simulink model "TST_RmtAPP_SelSig"  (R2016b)
settings: Solver=FixedStepDiscrete  StartTime=0.0  StopTime=simTime  FixedStep=sampleTime  RelTol=1e-3
values from neighbouring files (symbols this model uses):
  testCase = 1    [initTST_RmtAPP_SelSig_001.m]    (also in initTST_RmtAPP_SelSig_002.m = 2; initTST_RmtAPP_SelSig_003.m = 3; initTST_RmtAPP_SelSig_004.m = 4)
libraries: simulink x25, UnitTest_Lib x20
settings Model: Creator=liangyunbo  LastModifiedBy=liangyunbo
settings DebuggingCC: SignalRangeChecking=error

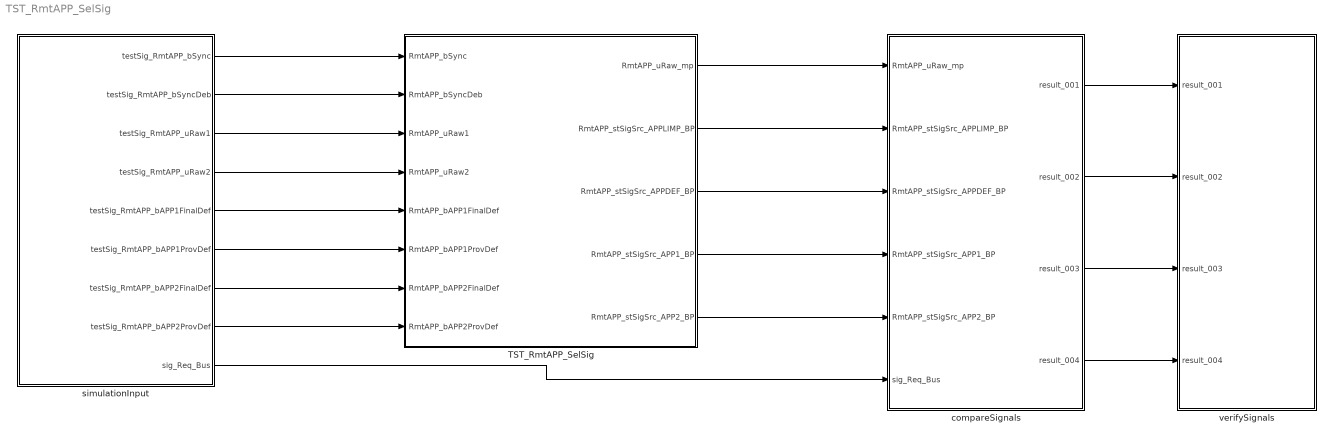
== system TST_RmtAPP_SelSig ==
  TST_RmtAPP_SelSig : Subsystem
  compareSignals : Subsystem
  simulationInput : Subsystem
  verifySignals : Subsystem
  wires:
  simulationInput/1(testSig_RmtAPP_bSync) -> TST_RmtAPP_SelSig/1(RmtAPP_bSync)
  simulationInput/2(testSig_RmtAPP_bSyncDeb) -> TST_RmtAPP_SelSig/2(RmtAPP_bSyncDeb)
  simulationInput/3(testSig_RmtAPP_uRaw1) -> TST_RmtAPP_SelSig/3(RmtAPP_uRaw1)
  simulationInput/4(testSig_RmtAPP_uRaw2) -> TST_RmtAPP_SelSig/4(RmtAPP_uRaw2)
  simulationInput/5(testSig_RmtAPP_bAPP1FinalDef) -> TST_RmtAPP_SelSig/5(RmtAPP_bAPP1FinalDef)
  simulationInput/6(testSig_RmtAPP_bAPP1ProvDef) -> TST_RmtAPP_SelSig/6(RmtAPP_bAPP1ProvDef)
  simulationInput/7(testSig_RmtAPP_bAPP2FinalDef) -> TST_RmtAPP_SelSig/7(RmtAPP_bAPP2FinalDef)
  simulationInput/8(testSig_RmtAPP_bAPP2ProvDef) -> TST_RmtAPP_SelSig/8(RmtAPP_bAPP2ProvDef)
  TST_RmtAPP_SelSig/1(RmtAPP_uRaw_mp) -> compareSignals/1(RmtAPP_uRaw_mp)
  TST_RmtAPP_SelSig/2(RmtAPP_stSigSrc_APPLIMP_BP) -> compareSignals/2(RmtAPP_stSigSrc_APPLIMP_BP)
  TST_RmtAPP_SelSig/3(RmtAPP_stSigSrc_APPDEF_BP) -> compareSignals/3(RmtAPP_stSigSrc_APPDEF_BP)
  TST_RmtAPP_SelSig/4(RmtAPP_stSigSrc_APP1_BP) -> compareSignals/4(RmtAPP_stSigSrc_APP1_BP)
  TST_RmtAPP_SelSig/5(RmtAPP_stSigSrc_APP2_BP) -> compareSignals/5(RmtAPP_stSigSrc_APP2_BP)
  simulationInput/9(sig_Req_Bus) -> compareSignals/6(sig_Req_Bus)
  compareSignals/1(result_001) -> verifySignals/1(result_001)
  compareSignals/2(result_002) -> verifySignals/2(result_002)
  compareSignals/3(result_003) -> verifySignals/3(result_003)
  compareSignals/4(result_004) -> verifySignals/4(result_004)

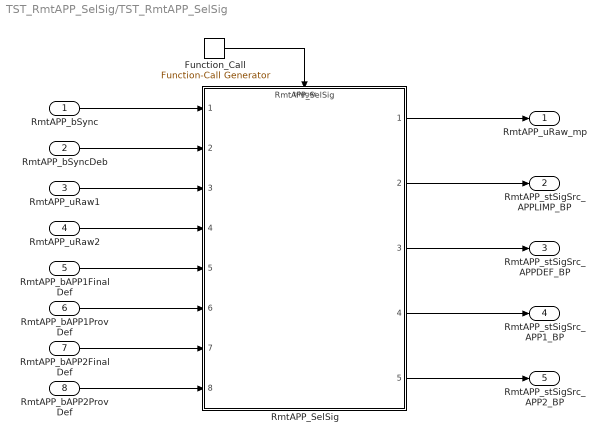
== system TST_RmtAPP_SelSig/TST_RmtAPP_SelSig ==
  RmtAPP_bSync : Inport
  RmtAPP_bSyncDeb : Inport  Port=2
  RmtAPP_uRaw1 : Inport  Port=3
  RmtAPP_uRaw2 : Inport  Port=4
  RmtAPP_bAPP1FinalDef : Inport  Port=5
  RmtAPP_bAPP1ProvDef : Inport  Port=6
  RmtAPP_bAPP2FinalDef : Inport  Port=7
  RmtAPP_bAPP2ProvDef : Inport  Port=8
  Function_Call : simulink/Ports & Subsystems/Function-Call Generator  sample_time=sampleTime  numberOfIterations=1
  RmtAPP_SelSig : ModelReference  ModelNameDialog=RmtAPP_SelSig  SimulationMode=Normal  ModelReferenceVersion=1.6  TriggerPortName=function  TriggerPortTriggerType=function-call  TriggerPortStatesWhenEnabling=held
  RmtAPP_uRaw_mp : Outport
  RmtAPP_stSigSrc_APPLIMP_BP : Outport  Port=2
  RmtAPP_stSigSrc_APPDEF_BP : Outport  Port=3
  RmtAPP_stSigSrc_APP1_BP : Outport  Port=4
  RmtAPP_stSigSrc_APP2_BP : Outport  Port=5
  wires:
  Function_Call/1 -> RmtAPP_SelSig/Trigger
  RmtAPP_bSync/1 -> RmtAPP_SelSig/1
  RmtAPP_bSyncDeb/1 -> RmtAPP_SelSig/2
  RmtAPP_uRaw1/1 -> RmtAPP_SelSig/3
  RmtAPP_uRaw2/1 -> RmtAPP_SelSig/4
  RmtAPP_bAPP1FinalDef/1 -> RmtAPP_SelSig/5
  RmtAPP_bAPP1ProvDef/1 -> RmtAPP_SelSig/6
  RmtAPP_bAPP2FinalDef/1 -> RmtAPP_SelSig/7
  RmtAPP_bAPP2ProvDef/1 -> RmtAPP_SelSig/8
  RmtAPP_SelSig/1 -> RmtAPP_uRaw_mp/1
  RmtAPP_SelSig/2 -> RmtAPP_stSigSrc_APPLIMP_BP/1
  RmtAPP_SelSig/3 -> RmtAPP_stSigSrc_APPDEF_BP/1
  RmtAPP_SelSig/4 -> RmtAPP_stSigSrc_APP1_BP/1
  RmtAPP_SelSig/5 -> RmtAPP_stSigSrc_APP2_BP/1

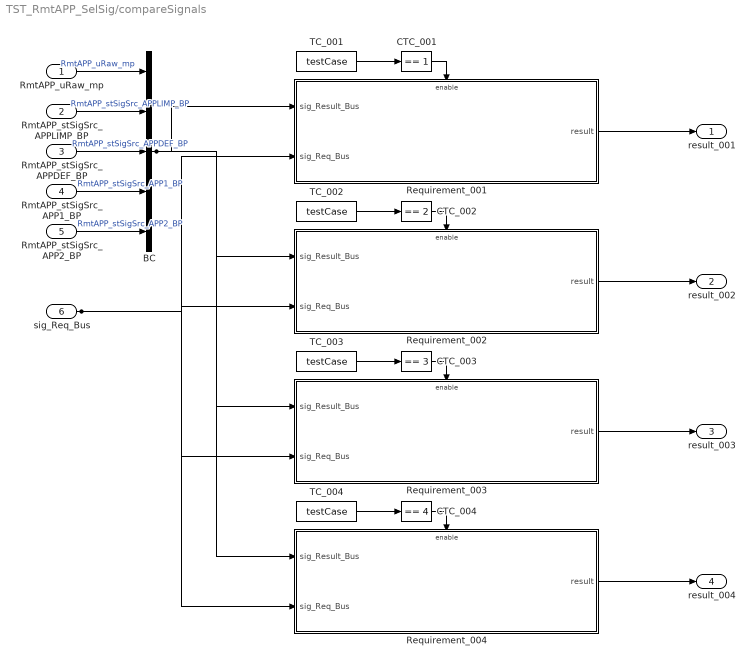
== system TST_RmtAPP_SelSig/compareSignals ==
  RmtAPP_uRaw_mp : Inport
  RmtAPP_stSigSrc_APPLIMP_BP : Inport  Port=2
  RmtAPP_stSigSrc_APPDEF_BP : Inport  Port=3
  RmtAPP_stSigSrc_APP1_BP : Inport  Port=4
  RmtAPP_stSigSrc_APP2_BP : Inport  Port=5
  sig_Req_Bus : Inport  Port=6
  BC : BusCreator  Inputs=5
  CTC_001 : simulink/Logic and Bit Operations/Compare To Constant  relop===  const=1  OutDataTypeStr=boolean
  CTC_002 : simulink/Logic and Bit Operations/Compare To Constant  relop===  const=2  OutDataTypeStr=boolean
  CTC_003 : simulink/Logic and Bit Operations/Compare To Constant  relop===  const=3  OutDataTypeStr=boolean
  CTC_004 : simulink/Logic and Bit Operations/Compare To Constant  relop===  const=4  OutDataTypeStr=boolean
  Requirement_001 : Subsystem
  Requirement_002 : Subsystem
  Requirement_003 : Subsystem
  Requirement_004 : Subsystem
  TC_001 : Constant  Value=testCase
  TC_002 : Constant  Value=testCase
  TC_003 : Constant  Value=testCase
  TC_004 : Constant  Value=testCase
  result_001 : Outport
  result_002 : Outport  Port=2
  result_003 : Outport  Port=3
  result_004 : Outport  Port=4
  wires:
  RmtAPP_uRaw_mp/1 -> BC/1  "RmtAPP_uRaw_mp"
  RmtAPP_stSigSrc_APPLIMP_BP/1 -> BC/2  "RmtAPP_stSigSrc_APPLIMP_BP"
  RmtAPP_stSigSrc_APPDEF_BP/1 -> BC/3  "RmtAPP_stSigSrc_APPDEF_BP"
  RmtAPP_stSigSrc_APP1_BP/1 -> BC/4  "RmtAPP_stSigSrc_APP1_BP"
  RmtAPP_stSigSrc_APP2_BP/1 -> BC/5  "RmtAPP_stSigSrc_APP2_BP"
  TC_001/1 -> CTC_001/1
  CTC_001/1 -> Requirement_001/Enable
  sig_Req_Bus/1 -> Requirement_001/2(sig_Req_Bus), Requirement_002/2(sig_Req_Bus), Requirement_003/2(sig_Req_Bus), Requirement_004/2(sig_Req_Bus)
  BC/1 -> Requirement_001/1(sig_Result_Bus), Requirement_002/1(sig_Result_Bus), Requirement_003/1(sig_Result_Bus), Requirement_004/1(sig_Result_Bus)
  Requirement_001/1(result) -> result_001/1
  TC_002/1 -> CTC_002/1
  CTC_002/1 -> Requirement_002/Enable
  Requirement_002/1(result) -> result_002/1
  TC_003/1 -> CTC_003/1
  CTC_003/1 -> Requirement_003/Enable
  Requirement_003/1(result) -> result_003/1
  TC_004/1 -> CTC_004/1
  CTC_004/1 -> Requirement_004/Enable
  Requirement_004/1(result) -> result_004/1

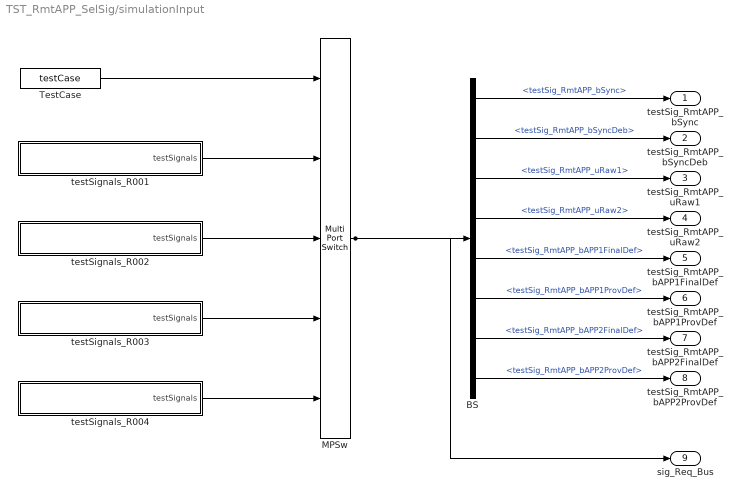
== system TST_RmtAPP_SelSig/simulationInput ==
  BS : BusSelector  OutputSignals=testSig_RmtAPP_bSync,testSig_RmtAPP_bSyncDeb,testSig_RmtAPP_uRaw1,testSig_RmtAPP_uRaw2,testSig_RmtAPP_bAPP1FinalDef,testSig_RmtAPP_bAPP1ProvDef,testSig_RmtAPP_bAPP2FinalDef,testSig_RmtAPP_bAPP2ProvDef
  MPSw : MultiPortSwitch  Inputs=4  SaturateOnIntegerOverflow=on  InputSameDT=on
  TestCase : Constant  Value=testCase
  testSignals_R001 : Subsystem
  testSignals_R002 : Subsystem
  testSignals_R003 : Subsystem
  testSignals_R004 : Subsystem
  testSig_RmtAPP_bSync : Outport
  testSig_RmtAPP_bSyncDeb : Outport  Port=2
  testSig_RmtAPP_uRaw1 : Outport  Port=3
  testSig_RmtAPP_uRaw2 : Outport  Port=4
  testSig_RmtAPP_bAPP1FinalDef : Outport  Port=5
  testSig_RmtAPP_bAPP1ProvDef : Outport  Port=6
  testSig_RmtAPP_bAPP2FinalDef : Outport  Port=7
  testSig_RmtAPP_bAPP2ProvDef : Outport  Port=8
  sig_Req_Bus : Outport  Port=9
  wires:
  BS/1 -> testSig_RmtAPP_bSync/1  "<testSig_RmtAPP_bSync>"
  BS/2 -> testSig_RmtAPP_bSyncDeb/1  "<testSig_RmtAPP_bSyncDeb>"
  BS/3 -> testSig_RmtAPP_uRaw1/1  "<testSig_RmtAPP_uRaw1>"
  BS/4 -> testSig_RmtAPP_uRaw2/1  "<testSig_RmtAPP_uRaw2>"
  BS/5 -> testSig_RmtAPP_bAPP1FinalDef/1  "<testSig_RmtAPP_bAPP1FinalDef>"
  BS/6 -> testSig_RmtAPP_bAPP1ProvDef/1  "<testSig_RmtAPP_bAPP1ProvDef>"
  BS/7 -> testSig_RmtAPP_bAPP2FinalDef/1  "<testSig_RmtAPP_bAPP2FinalDef>"
  BS/8 -> testSig_RmtAPP_bAPP2ProvDef/1  "<testSig_RmtAPP_bAPP2ProvDef>"
  MPSw/1 -> BS/1, sig_Req_Bus/1
  TestCase/1 -> MPSw/1
  testSignals_R001/1(testSignals) -> MPSw/2
  testSignals_R002/1(testSignals) -> MPSw/3
  testSignals_R003/1(testSignals) -> MPSw/4
  testSignals_R004/1(testSignals) -> MPSw/5

== system TST_RmtAPP_SelSig/verifySignals ==
  result_001 : Inport
  result_002 : Inport  Port=2
  result_003 : Inport  Port=3
  result_004 : Inport  Port=4
  Assertion_001 : Assertion  Enabled=off
  Assertion_002 : Assertion  Enabled=off
  Assertion_003 : Assertion  Enabled=off
  Assertion_004 : Assertion  Enabled=off
  wires:
  result_001/1 -> Assertion_001/1
  result_002/1 -> Assertion_002/1
  result_003/1 -> Assertion_003/1
  result_004/1 -> Assertion_004/1

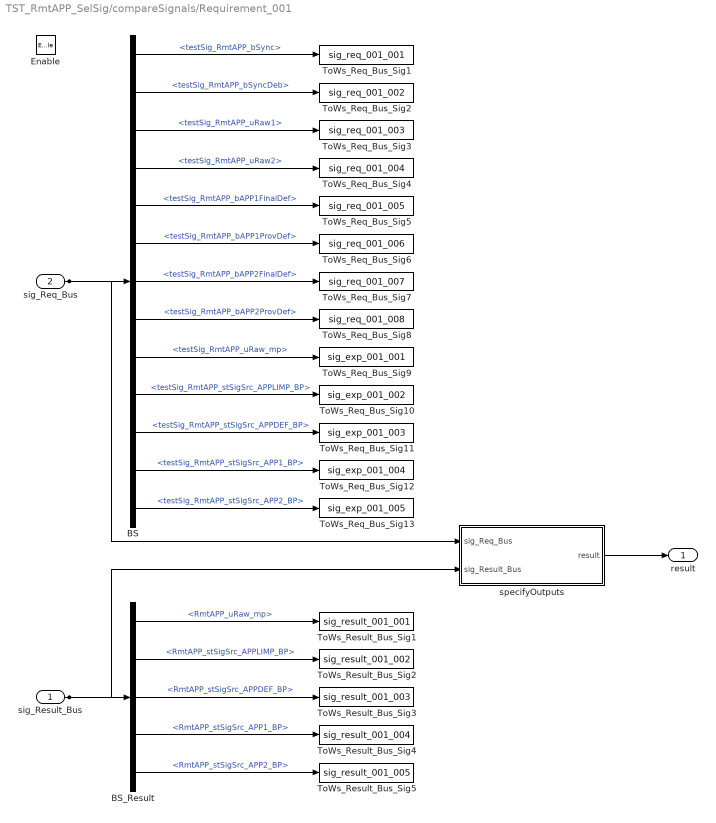
== system TST_RmtAPP_SelSig/compareSignals/Requirement_001 ==
  sig_Result_Bus : Inport
  sig_Req_Bus : Inport  Port=2
  Enable : EnablePort
  BS : BusSelector  OutputSignals=testSig_RmtAPP_bSync,testSig_RmtAPP_bSyncDeb,testSig_RmtAPP_uRaw1,testSig_RmtAPP_uRaw2,testSig_RmtAPP_bAPP1FinalDef,testSig_RmtAPP_bAPP1ProvDef,testSig_RmtAPP_bAPP2FinalDef,testSig_RmtAPP_bAPP2ProvDef,testSig_RmtAPP_uRaw_mp,testSig_RmtAPP_stSigSrc_APPLIMP_BP,testSig_RmtAPP_stSigSrc_APPDEF_BP,testSig_RmtAPP_stSigSrc_APP1_BP,testSig_RmtAPP_stSigSrc_APP2_BP
  BS_Result : BusSelector  OutputSignals=RmtAPP_uRaw_mp,RmtAPP_stSigSrc_APPLIMP_BP,RmtAPP_stSigSrc_APPDEF_BP,RmtAPP_stSigSrc_APP1_BP,RmtAPP_stSigSrc_APP2_BP
  ToWs_Req_Bus_Sig1 : ToWorkspace  VariableName=sig_req_001_001  SaveFormat=Structure With Time
  ToWs_Req_Bus_Sig10 : ToWorkspace  VariableName=sig_exp_001_002  SaveFormat=Structure With Time
  ToWs_Req_Bus_Sig11 : ToWorkspace  VariableName=sig_exp_001_003  SaveFormat=Structure With Time
  ToWs_Req_Bus_Sig12 : ToWorkspace  VariableName=sig_exp_001_004  SaveFormat=Structure With Time
  ToWs_Req_Bus_Sig13 : ToWorkspace  VariableName=sig_exp_001_005  SaveFormat=Structure With Time
  ToWs_Req_Bus_Sig2 : ToWorkspace  VariableName=sig_req_001_002  SaveFormat=Structure With Time
  ToWs_Req_Bus_Sig3 : ToWorkspace  VariableName=sig_req_001_003  SaveFormat=Structure With Time
  ToWs_Req_Bus_Sig4 : ToWorkspace  VariableName=sig_req_001_004  SaveFormat=Structure With Time
  ToWs_Req_Bus_Sig5 : ToWorkspace  VariableName=sig_req_001_005  SaveFormat=Structure With Time
  ToWs_Req_Bus_Sig6 : ToWorkspace  VariableName=sig_req_001_006  SaveFormat=Structure With Time
  ToWs_Req_Bus_Sig7 : ToWorkspace  VariableName=sig_req_001_007  SaveFormat=Structure With Time
  ToWs_Req_Bus_Sig8 : ToWorkspace  VariableName=sig_req_001_008  SaveFormat=Structure With Time
  ToWs_Req_Bus_Sig9 : ToWorkspace  VariableName=sig_exp_001_001  SaveFormat=Structure With Time
  ToWs_Result_Bus_Sig1 : ToWorkspace  VariableName=sig_result_001_001  SaveFormat=Structure With Time
  ToWs_Result_Bus_Sig2 : ToWorkspace  VariableName=sig_result_001_002  SaveFormat=Structure With Time
  ToWs_Result_Bus_Sig3 : ToWorkspace  VariableName=sig_result_001_003  SaveFormat=Structure With Time
  ToWs_Result_Bus_Sig4 : ToWorkspace  VariableName=sig_result_001_004  SaveFormat=Structure With Time
  ToWs_Result_Bus_Sig5 : ToWorkspace  VariableName=sig_result_001_005  SaveFormat=Structure With Time
  specifyOutputs : Subsystem
  result : Outport
  wires:
  sig_Req_Bus/1 -> BS/1, specifyOutputs/1(sig_Req_Bus)
  BS/1 -> ToWs_Req_Bus_Sig1/1  "<testSig_RmtAPP_bSync>"
  BS/2 -> ToWs_Req_Bus_Sig2/1  "<testSig_RmtAPP_bSyncDeb>"
  BS/3 -> ToWs_Req_Bus_Sig3/1  "<testSig_RmtAPP_uRaw1>"
  BS/4 -> ToWs_Req_Bus_Sig4/1  "<testSig_RmtAPP_uRaw2>"
  BS/5 -> ToWs_Req_Bus_Sig5/1  "<testSig_RmtAPP_bAPP1FinalDef>"
  BS/6 -> ToWs_Req_Bus_Sig6/1  "<testSig_RmtAPP_bAPP1ProvDef>"
  BS/7 -> ToWs_Req_Bus_Sig7/1  "<testSig_RmtAPP_bAPP2FinalDef>"
  BS/8 -> ToWs_Req_Bus_Sig8/1  "<testSig_RmtAPP_bAPP2ProvDef>"
  BS/9 -> ToWs_Req_Bus_Sig9/1  "<testSig_RmtAPP_uRaw_mp>"
  BS/10 -> ToWs_Req_Bus_Sig10/1  "<testSig_RmtAPP_stSigSrc_APPLIMP_BP>"
  BS/11 -> ToWs_Req_Bus_Sig11/1  "<testSig_RmtAPP_stSigSrc_APPDEF_BP>"
  BS/12 -> ToWs_Req_Bus_Sig12/1  "<testSig_RmtAPP_stSigSrc_APP1_BP>"
  BS/13 -> ToWs_Req_Bus_Sig13/1  "<testSig_RmtAPP_stSigSrc_APP2_BP>"
  sig_Result_Bus/1 -> BS_Result/1, specifyOutputs/2(sig_Result_Bus)
  BS_Result/1 -> ToWs_Result_Bus_Sig1/1  "<RmtAPP_uRaw_mp>"
  BS_Result/2 -> ToWs_Result_Bus_Sig2/1  "<RmtAPP_stSigSrc_APPLIMP_BP>"
  BS_Result/3 -> ToWs_Result_Bus_Sig3/1  "<RmtAPP_stSigSrc_APPDEF_BP>"
  BS_Result/4 -> ToWs_Result_Bus_Sig4/1  "<RmtAPP_stSigSrc_APP1_BP>"
  BS_Result/5 -> ToWs_Result_Bus_Sig5/1  "<RmtAPP_stSigSrc_APP2_BP>"
  specifyOutputs/1(result) -> result/1

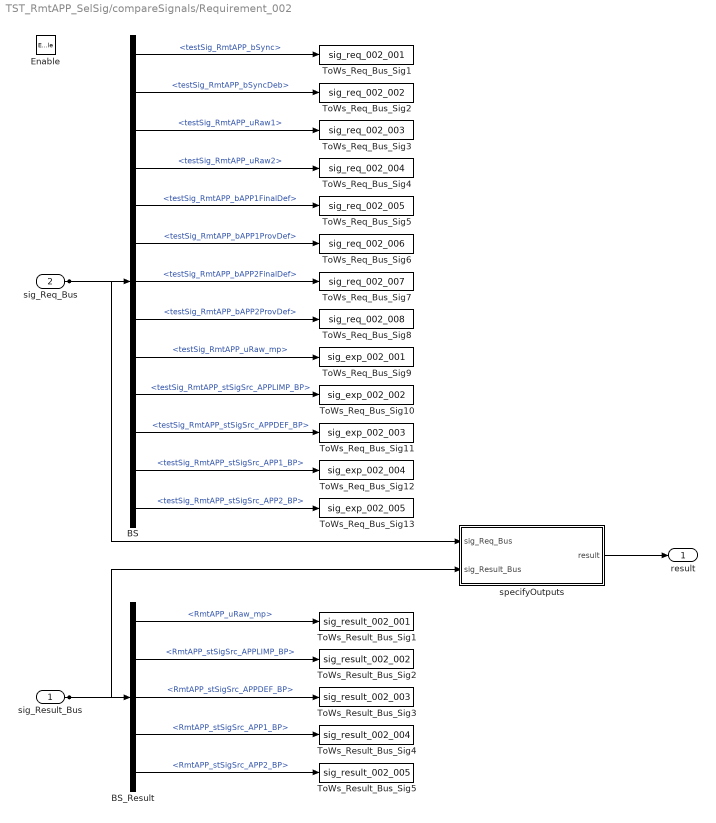
== system TST_RmtAPP_SelSig/compareSignals/Requirement_002 ==
  sig_Result_Bus : Inport
  sig_Req_Bus : Inport  Port=2
  Enable : EnablePort
  BS : BusSelector  OutputSignals=testSig_RmtAPP_bSync,testSig_RmtAPP_bSyncDeb,testSig_RmtAPP_uRaw1,testSig_RmtAPP_uRaw2,testSig_RmtAPP_bAPP1FinalDef,testSig_RmtAPP_bAPP1ProvDef,testSig_RmtAPP_bAPP2FinalDef,testSig_RmtAPP_bAPP2ProvDef,testSig_RmtAPP_uRaw_mp,testSig_RmtAPP_stSigSrc_APPLIMP_BP,testSig_RmtAPP_stSigSrc_APPDEF_BP,testSig_RmtAPP_stSigSrc_APP1_BP,testSig_RmtAPP_stSigSrc_APP2_BP
  BS_Result : BusSelector  OutputSignals=RmtAPP_uRaw_mp,RmtAPP_stSigSrc_APPLIMP_BP,RmtAPP_stSigSrc_APPDEF_BP,RmtAPP_stSigSrc_APP1_BP,RmtAPP_stSigSrc_APP2_BP
  ToWs_Req_Bus_Sig1 : ToWorkspace  VariableName=sig_req_002_001  SaveFormat=Structure With Time
  ToWs_Req_Bus_Sig10 : ToWorkspace  VariableName=sig_exp_002_002  SaveFormat=Structure With Time
  ToWs_Req_Bus_Sig11 : ToWorkspace  VariableName=sig_exp_002_003  SaveFormat=Structure With Time
  ToWs_Req_Bus_Sig12 : ToWorkspace  VariableName=sig_exp_002_004  SaveFormat=Structure With Time
  ToWs_Req_Bus_Sig13 : ToWorkspace  VariableName=sig_exp_002_005  SaveFormat=Structure With Time
  ToWs_Req_Bus_Sig2 : ToWorkspace  VariableName=sig_req_002_002  SaveFormat=Structure With Time
  ToWs_Req_Bus_Sig3 : ToWorkspace  VariableName=sig_req_002_003  SaveFormat=Structure With Time
  ToWs_Req_Bus_Sig4 : ToWorkspace  VariableName=sig_req_002_004  SaveFormat=Structure With Time
  ToWs_Req_Bus_Sig5 : ToWorkspace  VariableName=sig_req_002_005  SaveFormat=Structure With Time
  ToWs_Req_Bus_Sig6 : ToWorkspace  VariableName=sig_req_002_006  SaveFormat=Structure With Time
  ToWs_Req_Bus_Sig7 : ToWorkspace  VariableName=sig_req_002_007  SaveFormat=Structure With Time
  ToWs_Req_Bus_Sig8 : ToWorkspace  VariableName=sig_req_002_008  SaveFormat=Structure With Time
  ToWs_Req_Bus_Sig9 : ToWorkspace  VariableName=sig_exp_002_001  SaveFormat=Structure With Time
  ToWs_Result_Bus_Sig1 : ToWorkspace  VariableName=sig_result_002_001  SaveFormat=Structure With Time
  ToWs_Result_Bus_Sig2 : ToWorkspace  VariableName=sig_result_002_002  SaveFormat=Structure With Time
  ToWs_Result_Bus_Sig3 : ToWorkspace  VariableName=sig_result_002_003  SaveFormat=Structure With Time
  ToWs_Result_Bus_Sig4 : ToWorkspace  VariableName=sig_result_002_004  SaveFormat=Structure With Time
  ToWs_Result_Bus_Sig5 : ToWorkspace  VariableName=sig_result_002_005  SaveFormat=Structure With Time
  specifyOutputs : Subsystem
  result : Outport
  wires:
  sig_Req_Bus/1 -> BS/1, specifyOutputs/1(sig_Req_Bus)
  BS/1 -> ToWs_Req_Bus_Sig1/1  "<testSig_RmtAPP_bSync>"
  BS/2 -> ToWs_Req_Bus_Sig2/1  "<testSig_RmtAPP_bSyncDeb>"
  BS/3 -> ToWs_Req_Bus_Sig3/1  "<testSig_RmtAPP_uRaw1>"
  BS/4 -> ToWs_Req_Bus_Sig4/1  "<testSig_RmtAPP_uRaw2>"
  BS/5 -> ToWs_Req_Bus_Sig5/1  "<testSig_RmtAPP_bAPP1FinalDef>"
  BS/6 -> ToWs_Req_Bus_Sig6/1  "<testSig_RmtAPP_bAPP1ProvDef>"
  BS/7 -> ToWs_Req_Bus_Sig7/1  "<testSig_RmtAPP_bAPP2FinalDef>"
  BS/8 -> ToWs_Req_Bus_Sig8/1  "<testSig_RmtAPP_bAPP2ProvDef>"
  BS/9 -> ToWs_Req_Bus_Sig9/1  "<testSig_RmtAPP_uRaw_mp>"
  BS/10 -> ToWs_Req_Bus_Sig10/1  "<testSig_RmtAPP_stSigSrc_APPLIMP_BP>"
  BS/11 -> ToWs_Req_Bus_Sig11/1  "<testSig_RmtAPP_stSigSrc_APPDEF_BP>"
  BS/12 -> ToWs_Req_Bus_Sig12/1  "<testSig_RmtAPP_stSigSrc_APP1_BP>"
  BS/13 -> ToWs_Req_Bus_Sig13/1  "<testSig_RmtAPP_stSigSrc_APP2_BP>"
  sig_Result_Bus/1 -> BS_Result/1, specifyOutputs/2(sig_Result_Bus)
  BS_Result/1 -> ToWs_Result_Bus_Sig1/1  "<RmtAPP_uRaw_mp>"
  BS_Result/2 -> ToWs_Result_Bus_Sig2/1  "<RmtAPP_stSigSrc_APPLIMP_BP>"
  BS_Result/3 -> ToWs_Result_Bus_Sig3/1  "<RmtAPP_stSigSrc_APPDEF_BP>"
  BS_Result/4 -> ToWs_Result_Bus_Sig4/1  "<RmtAPP_stSigSrc_APP1_BP>"
  BS_Result/5 -> ToWs_Result_Bus_Sig5/1  "<RmtAPP_stSigSrc_APP2_BP>"
  specifyOutputs/1(result) -> result/1

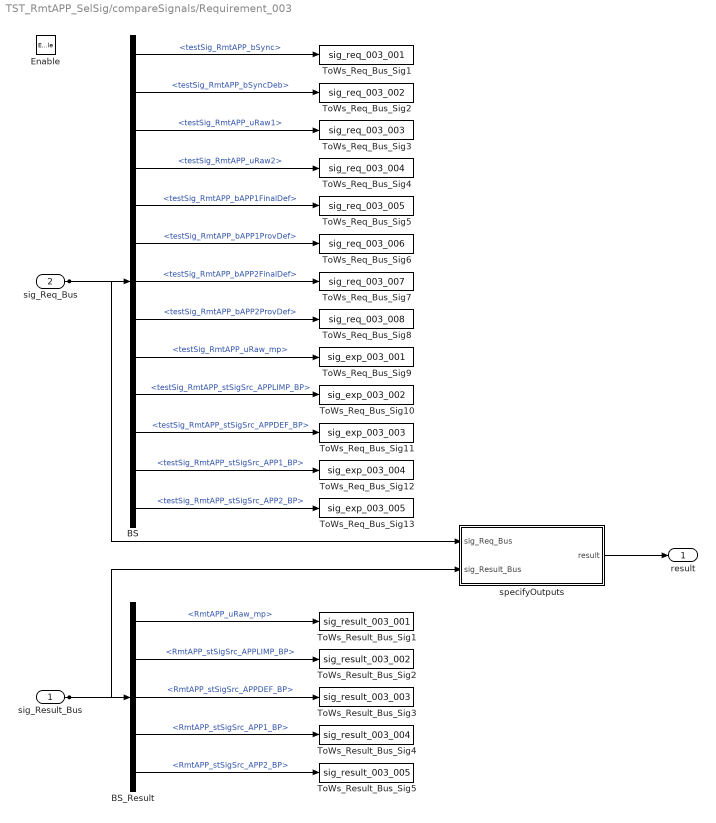
== system TST_RmtAPP_SelSig/compareSignals/Requirement_003 ==
  sig_Result_Bus : Inport
  sig_Req_Bus : Inport  Port=2
  Enable : EnablePort
  BS : BusSelector  OutputSignals=testSig_RmtAPP_bSync,testSig_RmtAPP_bSyncDeb,testSig_RmtAPP_uRaw1,testSig_RmtAPP_uRaw2,testSig_RmtAPP_bAPP1FinalDef,testSig_RmtAPP_bAPP1ProvDef,testSig_RmtAPP_bAPP2FinalDef,testSig_RmtAPP_bAPP2ProvDef,testSig_RmtAPP_uRaw_mp,testSig_RmtAPP_stSigSrc_APPLIMP_BP,testSig_RmtAPP_stSigSrc_APPDEF_BP,testSig_RmtAPP_stSigSrc_APP1_BP,testSig_RmtAPP_stSigSrc_APP2_BP
  BS_Result : BusSelector  OutputSignals=RmtAPP_uRaw_mp,RmtAPP_stSigSrc_APPLIMP_BP,RmtAPP_stSigSrc_APPDEF_BP,RmtAPP_stSigSrc_APP1_BP,RmtAPP_stSigSrc_APP2_BP
  ToWs_Req_Bus_Sig1 : ToWorkspace  VariableName=sig_req_003_001  SaveFormat=Structure With Time
  ToWs_Req_Bus_Sig10 : ToWorkspace  VariableName=sig_exp_003_002  SaveFormat=Structure With Time
  ToWs_Req_Bus_Sig11 : ToWorkspace  VariableName=sig_exp_003_003  SaveFormat=Structure With Time
  ToWs_Req_Bus_Sig12 : ToWorkspace  VariableName=sig_exp_003_004  SaveFormat=Structure With Time
  ToWs_Req_Bus_Sig13 : ToWorkspace  VariableName=sig_exp_003_005  SaveFormat=Structure With Time
  ToWs_Req_Bus_Sig2 : ToWorkspace  VariableName=sig_req_003_002  SaveFormat=Structure With Time
  ToWs_Req_Bus_Sig3 : ToWorkspace  VariableName=sig_req_003_003  SaveFormat=Structure With Time
  ToWs_Req_Bus_Sig4 : ToWorkspace  VariableName=sig_req_003_004  SaveFormat=Structure With Time
  ToWs_Req_Bus_Sig5 : ToWorkspace  VariableName=sig_req_003_005  SaveFormat=Structure With Time
  ToWs_Req_Bus_Sig6 : ToWorkspace  VariableName=sig_req_003_006  SaveFormat=Structure With Time
  ToWs_Req_Bus_Sig7 : ToWorkspace  VariableName=sig_req_003_007  SaveFormat=Structure With Time
  ToWs_Req_Bus_Sig8 : ToWorkspace  VariableName=sig_req_003_008  SaveFormat=Structure With Time
  ToWs_Req_Bus_Sig9 : ToWorkspace  VariableName=sig_exp_003_001  SaveFormat=Structure With Time
  ToWs_Result_Bus_Sig1 : ToWorkspace  VariableName=sig_result_003_001  SaveFormat=Structure With Time
  ToWs_Result_Bus_Sig2 : ToWorkspace  VariableName=sig_result_003_002  SaveFormat=Structure With Time
  ToWs_Result_Bus_Sig3 : ToWorkspace  VariableName=sig_result_003_003  SaveFormat=Structure With Time
  ToWs_Result_Bus_Sig4 : ToWorkspace  VariableName=sig_result_003_004  SaveFormat=Structure With Time
  ToWs_Result_Bus_Sig5 : ToWorkspace  VariableName=sig_result_003_005  SaveFormat=Structure With Time
  specifyOutputs : Subsystem
  result : Outport
  wires:
  sig_Req_Bus/1 -> BS/1, specifyOutputs/1(sig_Req_Bus)
  BS/1 -> ToWs_Req_Bus_Sig1/1  "<testSig_RmtAPP_bSync>"
  BS/2 -> ToWs_Req_Bus_Sig2/1  "<testSig_RmtAPP_bSyncDeb>"
  BS/3 -> ToWs_Req_Bus_Sig3/1  "<testSig_RmtAPP_uRaw1>"
  BS/4 -> ToWs_Req_Bus_Sig4/1  "<testSig_RmtAPP_uRaw2>"
  BS/5 -> ToWs_Req_Bus_Sig5/1  "<testSig_RmtAPP_bAPP1FinalDef>"
  BS/6 -> ToWs_Req_Bus_Sig6/1  "<testSig_RmtAPP_bAPP1ProvDef>"
  BS/7 -> ToWs_Req_Bus_Sig7/1  "<testSig_RmtAPP_bAPP2FinalDef>"
  BS/8 -> ToWs_Req_Bus_Sig8/1  "<testSig_RmtAPP_bAPP2ProvDef>"
  BS/9 -> ToWs_Req_Bus_Sig9/1  "<testSig_RmtAPP_uRaw_mp>"
  BS/10 -> ToWs_Req_Bus_Sig10/1  "<testSig_RmtAPP_stSigSrc_APPLIMP_BP>"
  BS/11 -> ToWs_Req_Bus_Sig11/1  "<testSig_RmtAPP_stSigSrc_APPDEF_BP>"
  BS/12 -> ToWs_Req_Bus_Sig12/1  "<testSig_RmtAPP_stSigSrc_APP1_BP>"
  BS/13 -> ToWs_Req_Bus_Sig13/1  "<testSig_RmtAPP_stSigSrc_APP2_BP>"
  sig_Result_Bus/1 -> BS_Result/1, specifyOutputs/2(sig_Result_Bus)
  BS_Result/1 -> ToWs_Result_Bus_Sig1/1  "<RmtAPP_uRaw_mp>"
  BS_Result/2 -> ToWs_Result_Bus_Sig2/1  "<RmtAPP_stSigSrc_APPLIMP_BP>"
  BS_Result/3 -> ToWs_Result_Bus_Sig3/1  "<RmtAPP_stSigSrc_APPDEF_BP>"
  BS_Result/4 -> ToWs_Result_Bus_Sig4/1  "<RmtAPP_stSigSrc_APP1_BP>"
  BS_Result/5 -> ToWs_Result_Bus_Sig5/1  "<RmtAPP_stSigSrc_APP2_BP>"
  specifyOutputs/1(result) -> result/1

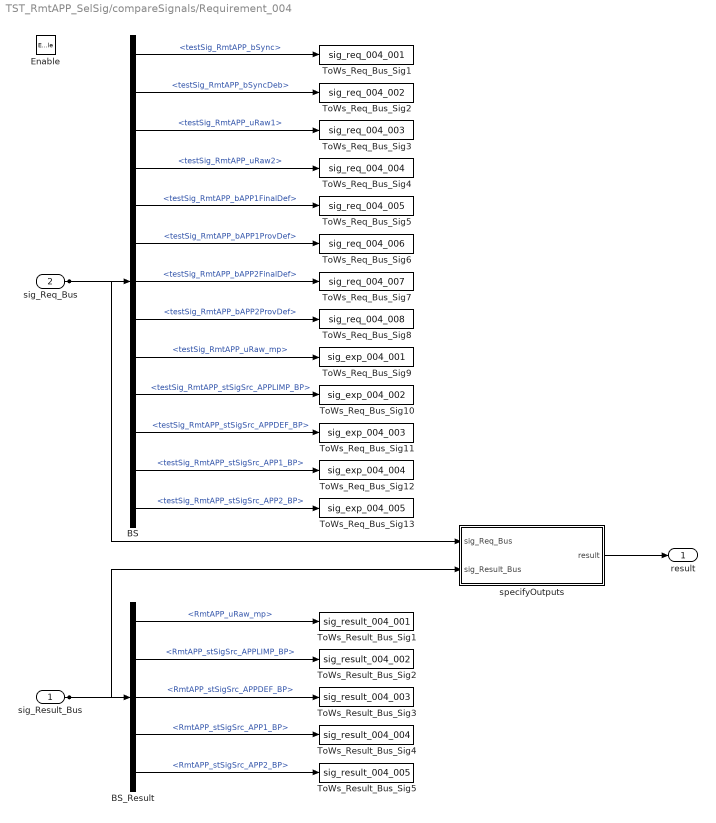
== system TST_RmtAPP_SelSig/compareSignals/Requirement_004 ==
  sig_Result_Bus : Inport
  sig_Req_Bus : Inport  Port=2
  Enable : EnablePort
  BS : BusSelector  OutputSignals=testSig_RmtAPP_bSync,testSig_RmtAPP_bSyncDeb,testSig_RmtAPP_uRaw1,testSig_RmtAPP_uRaw2,testSig_RmtAPP_bAPP1FinalDef,testSig_RmtAPP_bAPP1ProvDef,testSig_RmtAPP_bAPP2FinalDef,testSig_RmtAPP_bAPP2ProvDef,testSig_RmtAPP_uRaw_mp,testSig_RmtAPP_stSigSrc_APPLIMP_BP,testSig_RmtAPP_stSigSrc_APPDEF_BP,testSig_RmtAPP_stSigSrc_APP1_BP,testSig_RmtAPP_stSigSrc_APP2_BP
  BS_Result : BusSelector  OutputSignals=RmtAPP_uRaw_mp,RmtAPP_stSigSrc_APPLIMP_BP,RmtAPP_stSigSrc_APPDEF_BP,RmtAPP_stSigSrc_APP1_BP,RmtAPP_stSigSrc_APP2_BP
  ToWs_Req_Bus_Sig1 : ToWorkspace  VariableName=sig_req_004_001  SaveFormat=Structure With Time
  ToWs_Req_Bus_Sig10 : ToWorkspace  VariableName=sig_exp_004_002  SaveFormat=Structure With Time
  ToWs_Req_Bus_Sig11 : ToWorkspace  VariableName=sig_exp_004_003  SaveFormat=Structure With Time
  ToWs_Req_Bus_Sig12 : ToWorkspace  VariableName=sig_exp_004_004  SaveFormat=Structure With Time
  ToWs_Req_Bus_Sig13 : ToWorkspace  VariableName=sig_exp_004_005  SaveFormat=Structure With Time
  ToWs_Req_Bus_Sig2 : ToWorkspace  VariableName=sig_req_004_002  SaveFormat=Structure With Time
  ToWs_Req_Bus_Sig3 : ToWorkspace  VariableName=sig_req_004_003  SaveFormat=Structure With Time
  ToWs_Req_Bus_Sig4 : ToWorkspace  VariableName=sig_req_004_004  SaveFormat=Structure With Time
  ToWs_Req_Bus_Sig5 : ToWorkspace  VariableName=sig_req_004_005  SaveFormat=Structure With Time
  ToWs_Req_Bus_Sig6 : ToWorkspace  VariableName=sig_req_004_006  SaveFormat=Structure With Time
  ToWs_Req_Bus_Sig7 : ToWorkspace  VariableName=sig_req_004_007  SaveFormat=Structure With Time
  ToWs_Req_Bus_Sig8 : ToWorkspace  VariableName=sig_req_004_008  SaveFormat=Structure With Time
  ToWs_Req_Bus_Sig9 : ToWorkspace  VariableName=sig_exp_004_001  SaveFormat=Structure With Time
  ToWs_Result_Bus_Sig1 : ToWorkspace  VariableName=sig_result_004_001  SaveFormat=Structure With Time
  ToWs_Result_Bus_Sig2 : ToWorkspace  VariableName=sig_result_004_002  SaveFormat=Structure With Time
  ToWs_Result_Bus_Sig3 : ToWorkspace  VariableName=sig_result_004_003  SaveFormat=Structure With Time
  ToWs_Result_Bus_Sig4 : ToWorkspace  VariableName=sig_result_004_004  SaveFormat=Structure With Time
  ToWs_Result_Bus_Sig5 : ToWorkspace  VariableName=sig_result_004_005  SaveFormat=Structure With Time
  specifyOutputs : Subsystem
  result : Outport
  wires:
  sig_Req_Bus/1 -> BS/1, specifyOutputs/1(sig_Req_Bus)
  BS/1 -> ToWs_Req_Bus_Sig1/1  "<testSig_RmtAPP_bSync>"
  BS/2 -> ToWs_Req_Bus_Sig2/1  "<testSig_RmtAPP_bSyncDeb>"
  BS/3 -> ToWs_Req_Bus_Sig3/1  "<testSig_RmtAPP_uRaw1>"
  BS/4 -> ToWs_Req_Bus_Sig4/1  "<testSig_RmtAPP_uRaw2>"
  BS/5 -> ToWs_Req_Bus_Sig5/1  "<testSig_RmtAPP_bAPP1FinalDef>"
  BS/6 -> ToWs_Req_Bus_Sig6/1  "<testSig_RmtAPP_bAPP1ProvDef>"
  BS/7 -> ToWs_Req_Bus_Sig7/1  "<testSig_RmtAPP_bAPP2FinalDef>"
  BS/8 -> ToWs_Req_Bus_Sig8/1  "<testSig_RmtAPP_bAPP2ProvDef>"
  BS/9 -> ToWs_Req_Bus_Sig9/1  "<testSig_RmtAPP_uRaw_mp>"
  BS/10 -> ToWs_Req_Bus_Sig10/1  "<testSig_RmtAPP_stSigSrc_APPLIMP_BP>"
  BS/11 -> ToWs_Req_Bus_Sig11/1  "<testSig_RmtAPP_stSigSrc_APPDEF_BP>"
  BS/12 -> ToWs_Req_Bus_Sig12/1  "<testSig_RmtAPP_stSigSrc_APP1_BP>"
  BS/13 -> ToWs_Req_Bus_Sig13/1  "<testSig_RmtAPP_stSigSrc_APP2_BP>"
  sig_Result_Bus/1 -> BS_Result/1, specifyOutputs/2(sig_Result_Bus)
  BS_Result/1 -> ToWs_Result_Bus_Sig1/1  "<RmtAPP_uRaw_mp>"
  BS_Result/2 -> ToWs_Result_Bus_Sig2/1  "<RmtAPP_stSigSrc_APPLIMP_BP>"
  BS_Result/3 -> ToWs_Result_Bus_Sig3/1  "<RmtAPP_stSigSrc_APPDEF_BP>"
  BS_Result/4 -> ToWs_Result_Bus_Sig4/1  "<RmtAPP_stSigSrc_APP1_BP>"
  BS_Result/5 -> ToWs_Result_Bus_Sig5/1  "<RmtAPP_stSigSrc_APP2_BP>"
  specifyOutputs/1(result) -> result/1

== system TST_RmtAPP_SelSig/simulationInput/testSignals_R001 ==
  BC : BusCreator  Inputs=13
  spec_RmtAPP_bAPP1FinalDef : FromWorkspace  VariableName=testSig_RmtAPP_bAPP1FinalDef  Interpolate=off  OutputAfterFinalValue=Holding final value
  spec_RmtAPP_bAPP1ProvDef : FromWorkspace  VariableName=testSig_RmtAPP_bAPP1ProvDef  Interpolate=off  OutputAfterFinalValue=Holding final value
  spec_RmtAPP_bAPP2FinalDef : FromWorkspace  VariableName=testSig_RmtAPP_bAPP2FinalDef  Interpolate=off  OutputAfterFinalValue=Holding final value
  spec_RmtAPP_bAPP2ProvDef : FromWorkspace  VariableName=testSig_RmtAPP_bAPP2ProvDef  Interpolate=off  OutputAfterFinalValue=Holding final value
  spec_RmtAPP_bSync : FromWorkspace  VariableName=testSig_RmtAPP_bSync  Interpolate=off  OutputAfterFinalValue=Holding final value
  spec_RmtAPP_bSyncDeb : FromWorkspace  VariableName=testSig_RmtAPP_bSyncDeb  Interpolate=off  OutputAfterFinalValue=Holding final value
  spec_RmtAPP_stSigSrc_APP1_BP : FromWorkspace  VariableName=testSig_RmtAPP_stSigSrc_APP1_BP  Interpolate=off  OutputAfterFinalValue=Holding final value
  spec_RmtAPP_stSigSrc_APP2_BP : FromWorkspace  VariableName=testSig_RmtAPP_stSigSrc_APP2_BP  Interpolate=off  OutputAfterFinalValue=Holding final value
  spec_RmtAPP_stSigSrc_APPDEF_BP : FromWorkspace  VariableName=testSig_RmtAPP_stSigSrc_APPDEF_BP  Interpolate=off  OutputAfterFinalValue=Holding final value
  spec_RmtAPP_stSigSrc_APPLIMP_BP : FromWorkspace  VariableName=testSig_RmtAPP_stSigSrc_APPLIMP_BP  Interpolate=off  OutputAfterFinalValue=Holding final value
  spec_RmtAPP_uRaw1 : FromWorkspace  VariableName=testSig_RmtAPP_uRaw1  Interpolate=off  OutputAfterFinalValue=Holding final value
  spec_RmtAPP_uRaw2 : FromWorkspace  VariableName=testSig_RmtAPP_uRaw2  Interpolate=off  OutputAfterFinalValue=Holding final value
  spec_RmtAPP_uRaw_mp : FromWorkspace  VariableName=testSig_RmtAPP_uRaw_mp  Interpolate=off  OutputAfterFinalValue=Holding final value
  testSignals : Outport
  wires:
  BC/1 -> testSignals/1
  spec_RmtAPP_bSync/1 -> BC/1  "testSig_RmtAPP_bSync"
  spec_RmtAPP_bSyncDeb/1 -> BC/2  "testSig_RmtAPP_bSyncDeb"
  spec_RmtAPP_uRaw1/1 -> BC/3  "testSig_RmtAPP_uRaw1"
  spec_RmtAPP_uRaw2/1 -> BC/4  "testSig_RmtAPP_uRaw2"
  spec_RmtAPP_bAPP1FinalDef/1 -> BC/5  "testSig_RmtAPP_bAPP1FinalDef"
  spec_RmtAPP_bAPP1ProvDef/1 -> BC/6  "testSig_RmtAPP_bAPP1ProvDef"
  spec_RmtAPP_bAPP2FinalDef/1 -> BC/7  "testSig_RmtAPP_bAPP2FinalDef"
  spec_RmtAPP_bAPP2ProvDef/1 -> BC/8  "testSig_RmtAPP_bAPP2ProvDef"
  spec_RmtAPP_uRaw_mp/1 -> BC/9  "testSig_RmtAPP_uRaw_mp"
  spec_RmtAPP_stSigSrc_APPLIMP_BP/1 -> BC/10  "testSig_RmtAPP_stSigSrc_APPLIMP_BP"
  spec_RmtAPP_stSigSrc_APPDEF_BP/1 -> BC/11  "testSig_RmtAPP_stSigSrc_APPDEF_BP"
  spec_RmtAPP_stSigSrc_APP1_BP/1 -> BC/12  "testSig_RmtAPP_stSigSrc_APP1_BP"
  spec_RmtAPP_stSigSrc_APP2_BP/1 -> BC/13  "testSig_RmtAPP_stSigSrc_APP2_BP"

== system TST_RmtAPP_SelSig/simulationInput/testSignals_R002 ==
  BC : BusCreator  Inputs=13
  spec_RmtAPP_bAPP1FinalDef : FromWorkspace  VariableName=testSig_RmtAPP_bAPP1FinalDef  Interpolate=off  OutputAfterFinalValue=Holding final value
  spec_RmtAPP_bAPP1ProvDef : FromWorkspace  VariableName=testSig_RmtAPP_bAPP1ProvDef  Interpolate=off  OutputAfterFinalValue=Holding final value
  spec_RmtAPP_bAPP2FinalDef : FromWorkspace  VariableName=testSig_RmtAPP_bAPP2FinalDef  Interpolate=off  OutputAfterFinalValue=Holding final value
  spec_RmtAPP_bAPP2ProvDef : FromWorkspace  VariableName=testSig_RmtAPP_bAPP2ProvDef  Interpolate=off  OutputAfterFinalValue=Holding final value
  spec_RmtAPP_bSync : FromWorkspace  VariableName=testSig_RmtAPP_bSync  Interpolate=off  OutputAfterFinalValue=Holding final value
  spec_RmtAPP_bSyncDeb : FromWorkspace  VariableName=testSig_RmtAPP_bSyncDeb  Interpolate=off  OutputAfterFinalValue=Holding final value
  spec_RmtAPP_stSigSrc_APP1_BP : FromWorkspace  VariableName=testSig_RmtAPP_stSigSrc_APP1_BP  Interpolate=off  OutputAfterFinalValue=Holding final value
  spec_RmtAPP_stSigSrc_APP2_BP : FromWorkspace  VariableName=testSig_RmtAPP_stSigSrc_APP2_BP  Interpolate=off  OutputAfterFinalValue=Holding final value
  spec_RmtAPP_stSigSrc_APPDEF_BP : FromWorkspace  VariableName=testSig_RmtAPP_stSigSrc_APPDEF_BP  Interpolate=off  OutputAfterFinalValue=Holding final value
  spec_RmtAPP_stSigSrc_APPLIMP_BP : FromWorkspace  VariableName=testSig_RmtAPP_stSigSrc_APPLIMP_BP  Interpolate=off  OutputAfterFinalValue=Holding final value
  spec_RmtAPP_uRaw1 : FromWorkspace  VariableName=testSig_RmtAPP_uRaw1  Interpolate=off  OutputAfterFinalValue=Holding final value
  spec_RmtAPP_uRaw2 : FromWorkspace  VariableName=testSig_RmtAPP_uRaw2  Interpolate=off  OutputAfterFinalValue=Holding final value
  spec_RmtAPP_uRaw_mp : FromWorkspace  VariableName=testSig_RmtAPP_uRaw_mp  Interpolate=off  OutputAfterFinalValue=Holding final value
  testSignals : Outport
  wires:
  BC/1 -> testSignals/1
  spec_RmtAPP_bSync/1 -> BC/1  "testSig_RmtAPP_bSync"
  spec_RmtAPP_bSyncDeb/1 -> BC/2  "testSig_RmtAPP_bSyncDeb"
  spec_RmtAPP_uRaw1/1 -> BC/3  "testSig_RmtAPP_uRaw1"
  spec_RmtAPP_uRaw2/1 -> BC/4  "testSig_RmtAPP_uRaw2"
  spec_RmtAPP_bAPP1FinalDef/1 -> BC/5  "testSig_RmtAPP_bAPP1FinalDef"
  spec_RmtAPP_bAPP1ProvDef/1 -> BC/6  "testSig_RmtAPP_bAPP1ProvDef"
  spec_RmtAPP_bAPP2FinalDef/1 -> BC/7  "testSig_RmtAPP_bAPP2FinalDef"
  spec_RmtAPP_bAPP2ProvDef/1 -> BC/8  "testSig_RmtAPP_bAPP2ProvDef"
  spec_RmtAPP_uRaw_mp/1 -> BC/9  "testSig_RmtAPP_uRaw_mp"
  spec_RmtAPP_stSigSrc_APPLIMP_BP/1 -> BC/10  "testSig_RmtAPP_stSigSrc_APPLIMP_BP"
  spec_RmtAPP_stSigSrc_APPDEF_BP/1 -> BC/11  "testSig_RmtAPP_stSigSrc_APPDEF_BP"
  spec_RmtAPP_stSigSrc_APP1_BP/1 -> BC/12  "testSig_RmtAPP_stSigSrc_APP1_BP"
  spec_RmtAPP_stSigSrc_APP2_BP/1 -> BC/13  "testSig_RmtAPP_stSigSrc_APP2_BP"

== system TST_RmtAPP_SelSig/simulationInput/testSignals_R003 ==
  BC : BusCreator  Inputs=13
  spec_RmtAPP_bAPP1FinalDef : FromWorkspace  VariableName=testSig_RmtAPP_bAPP1FinalDef  Interpolate=off  OutputAfterFinalValue=Holding final value
  spec_RmtAPP_bAPP1ProvDef : FromWorkspace  VariableName=testSig_RmtAPP_bAPP1ProvDef  Interpolate=off  OutputAfterFinalValue=Holding final value
  spec_RmtAPP_bAPP2FinalDef : FromWorkspace  VariableName=testSig_RmtAPP_bAPP2FinalDef  Interpolate=off  OutputAfterFinalValue=Holding final value
  spec_RmtAPP_bAPP2ProvDef : FromWorkspace  VariableName=testSig_RmtAPP_bAPP2ProvDef  Interpolate=off  OutputAfterFinalValue=Holding final value
  spec_RmtAPP_bSync : FromWorkspace  VariableName=testSig_RmtAPP_bSync  Interpolate=off  OutputAfterFinalValue=Holding final value
  spec_RmtAPP_bSyncDeb : FromWorkspace  VariableName=testSig_RmtAPP_bSyncDeb  Interpolate=off  OutputAfterFinalValue=Holding final value
  spec_RmtAPP_stSigSrc_APP1_BP : FromWorkspace  VariableName=testSig_RmtAPP_stSigSrc_APP1_BP  Interpolate=off  OutputAfterFinalValue=Holding final value
  spec_RmtAPP_stSigSrc_APP2_BP : FromWorkspace  VariableName=testSig_RmtAPP_stSigSrc_APP2_BP  Interpolate=off  OutputAfterFinalValue=Holding final value
  spec_RmtAPP_stSigSrc_APPDEF_BP : FromWorkspace  VariableName=testSig_RmtAPP_stSigSrc_APPDEF_BP  Interpolate=off  OutputAfterFinalValue=Holding final value
  spec_RmtAPP_stSigSrc_APPLIMP_BP : FromWorkspace  VariableName=testSig_RmtAPP_stSigSrc_APPLIMP_BP  Interpolate=off  OutputAfterFinalValue=Holding final value
  spec_RmtAPP_uRaw1 : FromWorkspace  VariableName=testSig_RmtAPP_uRaw1  Interpolate=off  OutputAfterFinalValue=Holding final value
  spec_RmtAPP_uRaw2 : FromWorkspace  VariableName=testSig_RmtAPP_uRaw2  Interpolate=off  OutputAfterFinalValue=Holding final value
  spec_RmtAPP_uRaw_mp : FromWorkspace  VariableName=testSig_RmtAPP_uRaw_mp  Interpolate=off  OutputAfterFinalValue=Holding final value
  testSignals : Outport
  wires:
  BC/1 -> testSignals/1
  spec_RmtAPP_bSync/1 -> BC/1  "testSig_RmtAPP_bSync"
  spec_RmtAPP_bSyncDeb/1 -> BC/2  "testSig_RmtAPP_bSyncDeb"
  spec_RmtAPP_uRaw1/1 -> BC/3  "testSig_RmtAPP_uRaw1"
  spec_RmtAPP_uRaw2/1 -> BC/4  "testSig_RmtAPP_uRaw2"
  spec_RmtAPP_bAPP1FinalDef/1 -> BC/5  "testSig_RmtAPP_bAPP1FinalDef"
  spec_RmtAPP_bAPP1ProvDef/1 -> BC/6  "testSig_RmtAPP_bAPP1ProvDef"
  spec_RmtAPP_bAPP2FinalDef/1 -> BC/7  "testSig_RmtAPP_bAPP2FinalDef"
  spec_RmtAPP_bAPP2ProvDef/1 -> BC/8  "testSig_RmtAPP_bAPP2ProvDef"
  spec_RmtAPP_uRaw_mp/1 -> BC/9  "testSig_RmtAPP_uRaw_mp"
  spec_RmtAPP_stSigSrc_APPLIMP_BP/1 -> BC/10  "testSig_RmtAPP_stSigSrc_APPLIMP_BP"
  spec_RmtAPP_stSigSrc_APPDEF_BP/1 -> BC/11  "testSig_RmtAPP_stSigSrc_APPDEF_BP"
  spec_RmtAPP_stSigSrc_APP1_BP/1 -> BC/12  "testSig_RmtAPP_stSigSrc_APP1_BP"
  spec_RmtAPP_stSigSrc_APP2_BP/1 -> BC/13  "testSig_RmtAPP_stSigSrc_APP2_BP"

== system TST_RmtAPP_SelSig/simulationInput/testSignals_R004 ==
  BC : BusCreator  Inputs=13
  spec_RmtAPP_bAPP1FinalDef : FromWorkspace  VariableName=testSig_RmtAPP_bAPP1FinalDef  Interpolate=off  OutputAfterFinalValue=Holding final value
  spec_RmtAPP_bAPP1ProvDef : FromWorkspace  VariableName=testSig_RmtAPP_bAPP1ProvDef  Interpolate=off  OutputAfterFinalValue=Holding final value
  spec_RmtAPP_bAPP2FinalDef : FromWorkspace  VariableName=testSig_RmtAPP_bAPP2FinalDef  Interpolate=off  OutputAfterFinalValue=Holding final value
  spec_RmtAPP_bAPP2ProvDef : FromWorkspace  VariableName=testSig_RmtAPP_bAPP2ProvDef  Interpolate=off  OutputAfterFinalValue=Holding final value
  spec_RmtAPP_bSync : FromWorkspace  VariableName=testSig_RmtAPP_bSync  Interpolate=off  OutputAfterFinalValue=Holding final value
  spec_RmtAPP_bSyncDeb : FromWorkspace  VariableName=testSig_RmtAPP_bSyncDeb  Interpolate=off  OutputAfterFinalValue=Holding final value
  spec_RmtAPP_stSigSrc_APP1_BP : FromWorkspace  VariableName=testSig_RmtAPP_stSigSrc_APP1_BP  Interpolate=off  OutputAfterFinalValue=Holding final value
  spec_RmtAPP_stSigSrc_APP2_BP : FromWorkspace  VariableName=testSig_RmtAPP_stSigSrc_APP2_BP  Interpolate=off  OutputAfterFinalValue=Holding final value
  spec_RmtAPP_stSigSrc_APPDEF_BP : FromWorkspace  VariableName=testSig_RmtAPP_stSigSrc_APPDEF_BP  Interpolate=off  OutputAfterFinalValue=Holding final value
  spec_RmtAPP_stSigSrc_APPLIMP_BP : FromWorkspace  VariableName=testSig_RmtAPP_stSigSrc_APPLIMP_BP  Interpolate=off  OutputAfterFinalValue=Holding final value
  spec_RmtAPP_uRaw1 : FromWorkspace  VariableName=testSig_RmtAPP_uRaw1  Interpolate=off  OutputAfterFinalValue=Holding final value
  spec_RmtAPP_uRaw2 : FromWorkspace  VariableName=testSig_RmtAPP_uRaw2  Interpolate=off  OutputAfterFinalValue=Holding final value
  spec_RmtAPP_uRaw_mp : FromWorkspace  VariableName=testSig_RmtAPP_uRaw_mp  Interpolate=off  OutputAfterFinalValue=Holding final value
  testSignals : Outport
  wires:
  BC/1 -> testSignals/1
  spec_RmtAPP_bSync/1 -> BC/1  "testSig_RmtAPP_bSync"
  spec_RmtAPP_bSyncDeb/1 -> BC/2  "testSig_RmtAPP_bSyncDeb"
  spec_RmtAPP_uRaw1/1 -> BC/3  "testSig_RmtAPP_uRaw1"
  spec_RmtAPP_uRaw2/1 -> BC/4  "testSig_RmtAPP_uRaw2"
  spec_RmtAPP_bAPP1FinalDef/1 -> BC/5  "testSig_RmtAPP_bAPP1FinalDef"
  spec_RmtAPP_bAPP1ProvDef/1 -> BC/6  "testSig_RmtAPP_bAPP1ProvDef"
  spec_RmtAPP_bAPP2FinalDef/1 -> BC/7  "testSig_RmtAPP_bAPP2FinalDef"
  spec_RmtAPP_bAPP2ProvDef/1 -> BC/8  "testSig_RmtAPP_bAPP2ProvDef"
  spec_RmtAPP_uRaw_mp/1 -> BC/9  "testSig_RmtAPP_uRaw_mp"
  spec_RmtAPP_stSigSrc_APPLIMP_BP/1 -> BC/10  "testSig_RmtAPP_stSigSrc_APPLIMP_BP"
  spec_RmtAPP_stSigSrc_APPDEF_BP/1 -> BC/11  "testSig_RmtAPP_stSigSrc_APPDEF_BP"
  spec_RmtAPP_stSigSrc_APP1_BP/1 -> BC/12  "testSig_RmtAPP_stSigSrc_APP1_BP"
  spec_RmtAPP_stSigSrc_APP2_BP/1 -> BC/13  "testSig_RmtAPP_stSigSrc_APP2_BP"

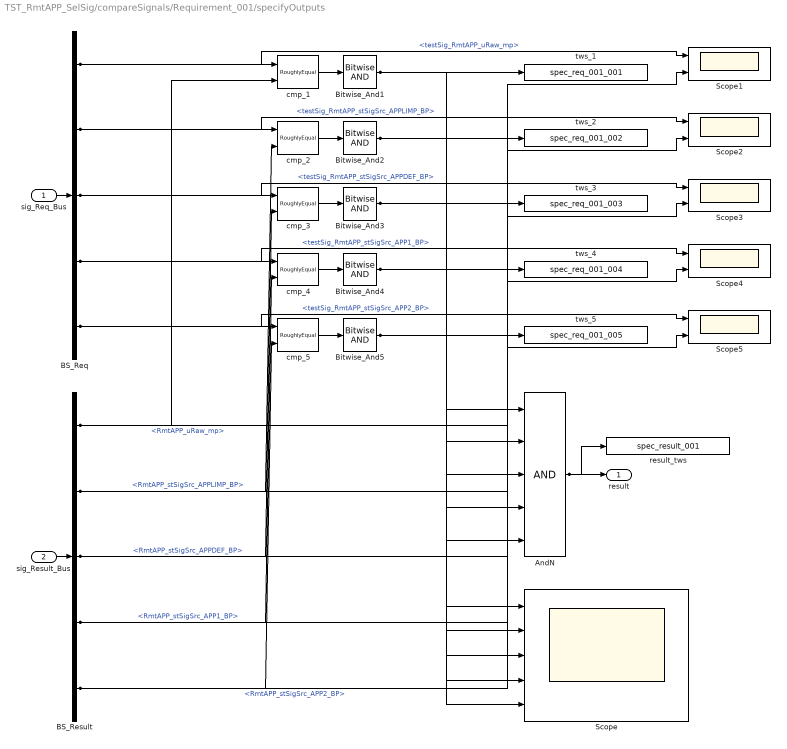
== system TST_RmtAPP_SelSig/compareSignals/Requirement_001/specifyOutputs ==
  sig_Req_Bus : Inport
  sig_Result_Bus : Inport  Port=2
  AndN : Logic  Inputs=5
  BS_Req : BusSelector  OutputSignals=testSig_RmtAPP_uRaw_mp,testSig_RmtAPP_stSigSrc_APPLIMP_BP,testSig_RmtAPP_stSigSrc_APPDEF_BP,testSig_RmtAPP_stSigSrc_APP1_BP,testSig_RmtAPP_stSigSrc_APP2_BP
  BS_Result : BusSelector  OutputSignals=RmtAPP_uRaw_mp,RmtAPP_stSigSrc_APPLIMP_BP,RmtAPP_stSigSrc_APPDEF_BP,RmtAPP_stSigSrc_APP1_BP,RmtAPP_stSigSrc_APP2_BP
  Bitwise_And{1..5} (5 alike) : simulink/Logic and Bit Operations/Bitwise Operator  logicop=AND  UseBitMask=off  BitMask=bin2dec('11011001')  BitMaskRealWorld=Stored Integer
  Scope : Scope  NumInputPorts=5
  Scope{1..5} (5 alike) : Scope  NumInputPorts=2
  cmp_{1..5} (5 alike) : UnitTest_Lib/RoughlyEqual  slope=0.1
  result_tws : ToWorkspace  VariableName=spec_result_001
  tws_1 : ToWorkspace  VariableName=spec_req_001_001
  tws_2 : ToWorkspace  VariableName=spec_req_001_002
  tws_3 : ToWorkspace  VariableName=spec_req_001_003
  tws_4 : ToWorkspace  VariableName=spec_req_001_004
  tws_5 : ToWorkspace  VariableName=spec_req_001_005
  result : Outport
  wires:
  sig_Req_Bus/1 -> BS_Req/1
  sig_Result_Bus/1 -> BS_Result/1
  AndN/1 -> result/1, result_tws/1
  BS_Req/1 -> cmp_1/1, Scope1/1  "<testSig_RmtAPP_uRaw_mp>"
  BS_Result/1 -> cmp_1/2, Scope1/2  "<RmtAPP_uRaw_mp>"
  cmp_1/1 -> Bitwise_And1/1
  Bitwise_And1/1 -> tws_1/1, AndN/1, Scope/1
  BS_Req/2 -> cmp_2/1, Scope2/1  "<testSig_RmtAPP_stSigSrc_APPLIMP_BP>"
  BS_Result/2 -> cmp_2/2, Scope2/2  "<RmtAPP_stSigSrc_APPLIMP_BP>"
  cmp_2/1 -> Bitwise_And2/1
  Bitwise_And2/1 -> tws_2/1, AndN/2, Scope/2
  BS_Req/3 -> cmp_3/1, Scope3/1  "<testSig_RmtAPP_stSigSrc_APPDEF_BP>"
  BS_Result/3 -> cmp_3/2, Scope3/2  "<RmtAPP_stSigSrc_APPDEF_BP>"
  cmp_3/1 -> Bitwise_And3/1
  Bitwise_And3/1 -> tws_3/1, AndN/3, Scope/3
  BS_Req/4 -> cmp_4/1, Scope4/1  "<testSig_RmtAPP_stSigSrc_APP1_BP>"
  BS_Result/4 -> cmp_4/2, Scope4/2  "<RmtAPP_stSigSrc_APP1_BP>"
  cmp_4/1 -> Bitwise_And4/1
  Bitwise_And4/1 -> tws_4/1, AndN/4, Scope/4
  BS_Req/5 -> cmp_5/1, Scope5/1  "<testSig_RmtAPP_stSigSrc_APP2_BP>"
  BS_Result/5 -> cmp_5/2, Scope5/2  "<RmtAPP_stSigSrc_APP2_BP>"
  cmp_5/1 -> Bitwise_And5/1
  Bitwise_And5/1 -> tws_5/1, AndN/5, Scope/5

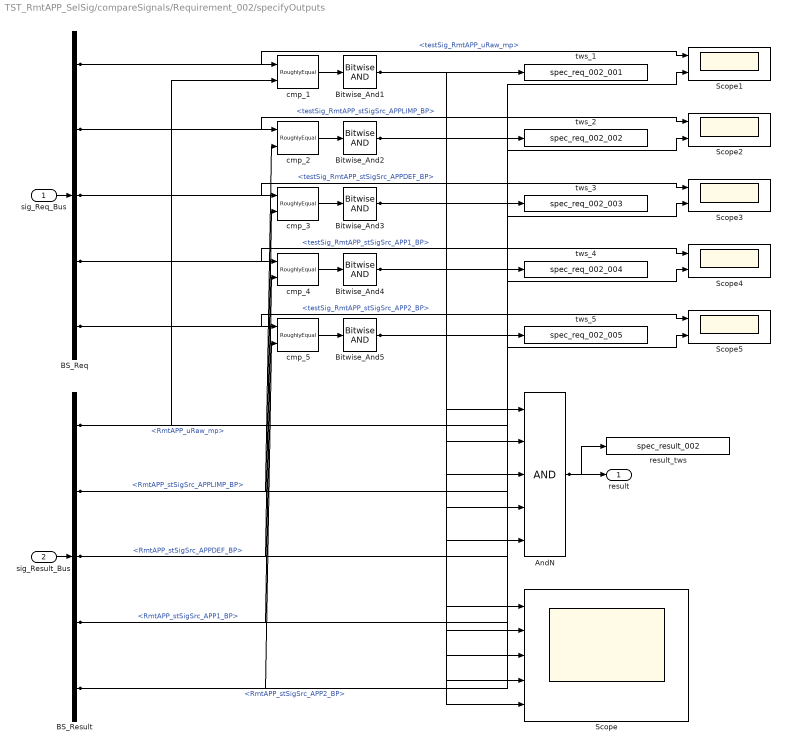
== system TST_RmtAPP_SelSig/compareSignals/Requirement_002/specifyOutputs ==
  sig_Req_Bus : Inport
  sig_Result_Bus : Inport  Port=2
  AndN : Logic  Inputs=5
  BS_Req : BusSelector  OutputSignals=testSig_RmtAPP_uRaw_mp,testSig_RmtAPP_stSigSrc_APPLIMP_BP,testSig_RmtAPP_stSigSrc_APPDEF_BP,testSig_RmtAPP_stSigSrc_APP1_BP,testSig_RmtAPP_stSigSrc_APP2_BP
  BS_Result : BusSelector  OutputSignals=RmtAPP_uRaw_mp,RmtAPP_stSigSrc_APPLIMP_BP,RmtAPP_stSigSrc_APPDEF_BP,RmtAPP_stSigSrc_APP1_BP,RmtAPP_stSigSrc_APP2_BP
  Bitwise_And{1..5} (5 alike) : simulink/Logic and Bit Operations/Bitwise Operator  logicop=AND  UseBitMask=off  BitMask=bin2dec('11011001')  BitMaskRealWorld=Stored Integer
  Scope : Scope  NumInputPorts=5
  Scope{1..5} (5 alike) : Scope  NumInputPorts=2
  cmp_{1..5} (5 alike) : UnitTest_Lib/RoughlyEqual  slope=0.1
  result_tws : ToWorkspace  VariableName=spec_result_002
  tws_1 : ToWorkspace  VariableName=spec_req_002_001
  tws_2 : ToWorkspace  VariableName=spec_req_002_002
  tws_3 : ToWorkspace  VariableName=spec_req_002_003
  tws_4 : ToWorkspace  VariableName=spec_req_002_004
  tws_5 : ToWorkspace  VariableName=spec_req_002_005
  result : Outport
  wires:
  sig_Req_Bus/1 -> BS_Req/1
  sig_Result_Bus/1 -> BS_Result/1
  AndN/1 -> result/1, result_tws/1
  BS_Req/1 -> cmp_1/1, Scope1/1  "<testSig_RmtAPP_uRaw_mp>"
  BS_Result/1 -> cmp_1/2, Scope1/2  "<RmtAPP_uRaw_mp>"
  cmp_1/1 -> Bitwise_And1/1
  Bitwise_And1/1 -> tws_1/1, AndN/1, Scope/1
  BS_Req/2 -> cmp_2/1, Scope2/1  "<testSig_RmtAPP_stSigSrc_APPLIMP_BP>"
  BS_Result/2 -> cmp_2/2, Scope2/2  "<RmtAPP_stSigSrc_APPLIMP_BP>"
  cmp_2/1 -> Bitwise_And2/1
  Bitwise_And2/1 -> tws_2/1, AndN/2, Scope/2
  BS_Req/3 -> cmp_3/1, Scope3/1  "<testSig_RmtAPP_stSigSrc_APPDEF_BP>"
  BS_Result/3 -> cmp_3/2, Scope3/2  "<RmtAPP_stSigSrc_APPDEF_BP>"
  cmp_3/1 -> Bitwise_And3/1
  Bitwise_And3/1 -> tws_3/1, AndN/3, Scope/3
  BS_Req/4 -> cmp_4/1, Scope4/1  "<testSig_RmtAPP_stSigSrc_APP1_BP>"
  BS_Result/4 -> cmp_4/2, Scope4/2  "<RmtAPP_stSigSrc_APP1_BP>"
  cmp_4/1 -> Bitwise_And4/1
  Bitwise_And4/1 -> tws_4/1, AndN/4, Scope/4
  BS_Req/5 -> cmp_5/1, Scope5/1  "<testSig_RmtAPP_stSigSrc_APP2_BP>"
  BS_Result/5 -> cmp_5/2, Scope5/2  "<RmtAPP_stSigSrc_APP2_BP>"
  cmp_5/1 -> Bitwise_And5/1
  Bitwise_And5/1 -> tws_5/1, AndN/5, Scope/5

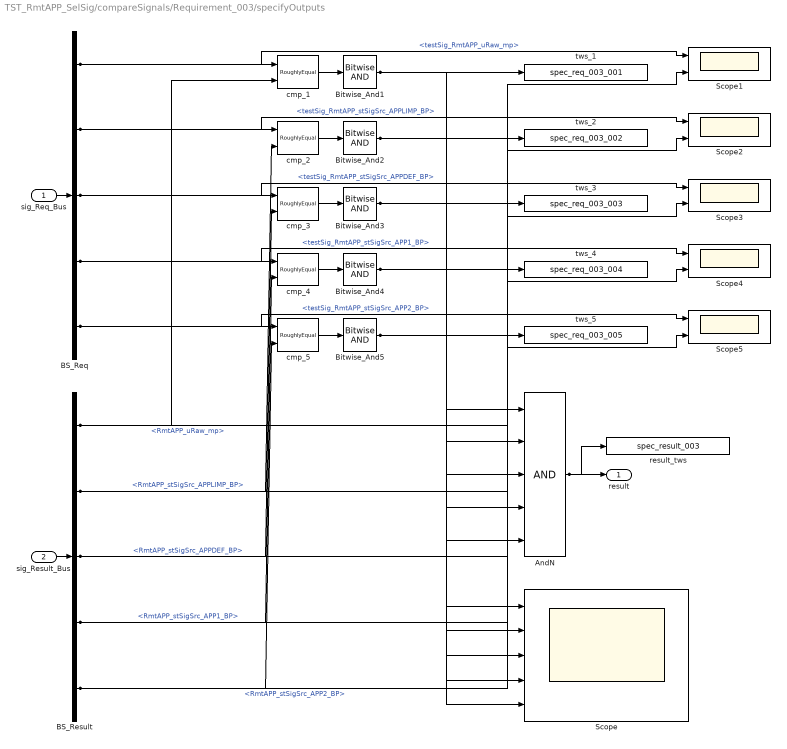
== system TST_RmtAPP_SelSig/compareSignals/Requirement_003/specifyOutputs ==
  sig_Req_Bus : Inport
  sig_Result_Bus : Inport  Port=2
  AndN : Logic  Inputs=5
  BS_Req : BusSelector  OutputSignals=testSig_RmtAPP_uRaw_mp,testSig_RmtAPP_stSigSrc_APPLIMP_BP,testSig_RmtAPP_stSigSrc_APPDEF_BP,testSig_RmtAPP_stSigSrc_APP1_BP,testSig_RmtAPP_stSigSrc_APP2_BP
  BS_Result : BusSelector  OutputSignals=RmtAPP_uRaw_mp,RmtAPP_stSigSrc_APPLIMP_BP,RmtAPP_stSigSrc_APPDEF_BP,RmtAPP_stSigSrc_APP1_BP,RmtAPP_stSigSrc_APP2_BP
  Bitwise_And{1..5} (5 alike) : simulink/Logic and Bit Operations/Bitwise Operator  logicop=AND  UseBitMask=off  BitMask=bin2dec('11011001')  BitMaskRealWorld=Stored Integer
  Scope : Scope  NumInputPorts=5
  Scope{1..5} (5 alike) : Scope  NumInputPorts=2
  cmp_{1..5} (5 alike) : UnitTest_Lib/RoughlyEqual  slope=0.1
  result_tws : ToWorkspace  VariableName=spec_result_003
  tws_1 : ToWorkspace  VariableName=spec_req_003_001
  tws_2 : ToWorkspace  VariableName=spec_req_003_002
  tws_3 : ToWorkspace  VariableName=spec_req_003_003
  tws_4 : ToWorkspace  VariableName=spec_req_003_004
  tws_5 : ToWorkspace  VariableName=spec_req_003_005
  result : Outport
  wires:
  sig_Req_Bus/1 -> BS_Req/1
  sig_Result_Bus/1 -> BS_Result/1
  AndN/1 -> result/1, result_tws/1
  BS_Req/1 -> cmp_1/1, Scope1/1  "<testSig_RmtAPP_uRaw_mp>"
  BS_Result/1 -> cmp_1/2, Scope1/2  "<RmtAPP_uRaw_mp>"
  cmp_1/1 -> Bitwise_And1/1
  Bitwise_And1/1 -> tws_1/1, AndN/1, Scope/1
  BS_Req/2 -> cmp_2/1, Scope2/1  "<testSig_RmtAPP_stSigSrc_APPLIMP_BP>"
  BS_Result/2 -> cmp_2/2, Scope2/2  "<RmtAPP_stSigSrc_APPLIMP_BP>"
  cmp_2/1 -> Bitwise_And2/1
  Bitwise_And2/1 -> tws_2/1, AndN/2, Scope/2
  BS_Req/3 -> cmp_3/1, Scope3/1  "<testSig_RmtAPP_stSigSrc_APPDEF_BP>"
  BS_Result/3 -> cmp_3/2, Scope3/2  "<RmtAPP_stSigSrc_APPDEF_BP>"
  cmp_3/1 -> Bitwise_And3/1
  Bitwise_And3/1 -> tws_3/1, AndN/3, Scope/3
  BS_Req/4 -> cmp_4/1, Scope4/1  "<testSig_RmtAPP_stSigSrc_APP1_BP>"
  BS_Result/4 -> cmp_4/2, Scope4/2  "<RmtAPP_stSigSrc_APP1_BP>"
  cmp_4/1 -> Bitwise_And4/1
  Bitwise_And4/1 -> tws_4/1, AndN/4, Scope/4
  BS_Req/5 -> cmp_5/1, Scope5/1  "<testSig_RmtAPP_stSigSrc_APP2_BP>"
  BS_Result/5 -> cmp_5/2, Scope5/2  "<RmtAPP_stSigSrc_APP2_BP>"
  cmp_5/1 -> Bitwise_And5/1
  Bitwise_And5/1 -> tws_5/1, AndN/5, Scope/5

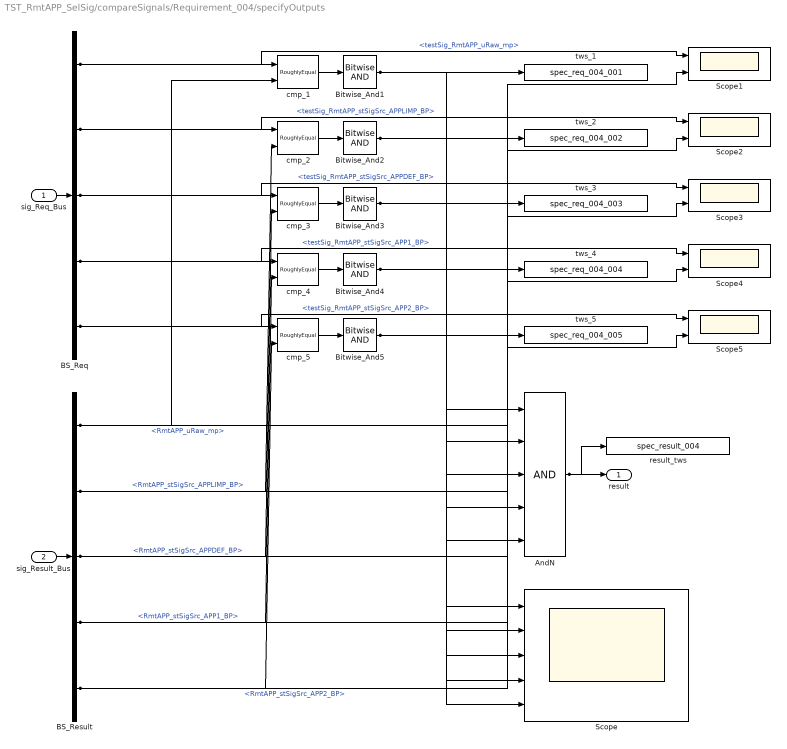
== system TST_RmtAPP_SelSig/compareSignals/Requirement_004/specifyOutputs ==
  sig_Req_Bus : Inport
  sig_Result_Bus : Inport  Port=2
  AndN : Logic  Inputs=5
  BS_Req : BusSelector  OutputSignals=testSig_RmtAPP_uRaw_mp,testSig_RmtAPP_stSigSrc_APPLIMP_BP,testSig_RmtAPP_stSigSrc_APPDEF_BP,testSig_RmtAPP_stSigSrc_APP1_BP,testSig_RmtAPP_stSigSrc_APP2_BP
  BS_Result : BusSelector  OutputSignals=RmtAPP_uRaw_mp,RmtAPP_stSigSrc_APPLIMP_BP,RmtAPP_stSigSrc_APPDEF_BP,RmtAPP_stSigSrc_APP1_BP,RmtAPP_stSigSrc_APP2_BP
  Bitwise_And{1..5} (5 alike) : simulink/Logic and Bit Operations/Bitwise Operator  logicop=AND  UseBitMask=off  BitMask=bin2dec('11011001')  BitMaskRealWorld=Stored Integer
  Scope : Scope  NumInputPorts=5
  Scope{1..5} (5 alike) : Scope  NumInputPorts=2
  cmp_{1..5} (5 alike) : UnitTest_Lib/RoughlyEqual  slope=0.1
  result_tws : ToWorkspace  VariableName=spec_result_004
  tws_1 : ToWorkspace  VariableName=spec_req_004_001
  tws_2 : ToWorkspace  VariableName=spec_req_004_002
  tws_3 : ToWorkspace  VariableName=spec_req_004_003
  tws_4 : ToWorkspace  VariableName=spec_req_004_004
  tws_5 : ToWorkspace  VariableName=spec_req_004_005
  result : Outport
  wires:
  sig_Req_Bus/1 -> BS_Req/1
  sig_Result_Bus/1 -> BS_Result/1
  AndN/1 -> result/1, result_tws/1
  BS_Req/1 -> cmp_1/1, Scope1/1  "<testSig_RmtAPP_uRaw_mp>"
  BS_Result/1 -> cmp_1/2, Scope1/2  "<RmtAPP_uRaw_mp>"
  cmp_1/1 -> Bitwise_And1/1
  Bitwise_And1/1 -> tws_1/1, AndN/1, Scope/1
  BS_Req/2 -> cmp_2/1, Scope2/1  "<testSig_RmtAPP_stSigSrc_APPLIMP_BP>"
  BS_Result/2 -> cmp_2/2, Scope2/2  "<RmtAPP_stSigSrc_APPLIMP_BP>"
  cmp_2/1 -> Bitwise_And2/1
  Bitwise_And2/1 -> tws_2/1, AndN/2, Scope/2
  BS_Req/3 -> cmp_3/1, Scope3/1  "<testSig_RmtAPP_stSigSrc_APPDEF_BP>"
  BS_Result/3 -> cmp_3/2, Scope3/2  "<RmtAPP_stSigSrc_APPDEF_BP>"
  cmp_3/1 -> Bitwise_And3/1
  Bitwise_And3/1 -> tws_3/1, AndN/3, Scope/3
  BS_Req/4 -> cmp_4/1, Scope4/1  "<testSig_RmtAPP_stSigSrc_APP1_BP>"
  BS_Result/4 -> cmp_4/2, Scope4/2  "<RmtAPP_stSigSrc_APP1_BP>"
  cmp_4/1 -> Bitwise_And4/1
  Bitwise_And4/1 -> tws_4/1, AndN/4, Scope/4
  BS_Req/5 -> cmp_5/1, Scope5/1  "<testSig_RmtAPP_stSigSrc_APP2_BP>"
  BS_Result/5 -> cmp_5/2, Scope5/2  "<RmtAPP_stSigSrc_APP2_BP>"
  cmp_5/1 -> Bitwise_And5/1
  Bitwise_And5/1 -> tws_5/1, AndN/5, Scope/5
